simulink model "Part1_Developing_a_Vehicle_Model_in_Simulink_from_Scratch"  (R2021a)
settings: Solver=VariableStepAuto  StartTime=0.0  StopTime=10.0  RelTol=1e-3
settings Model: Creator=QZHAN112  LastModifiedBy=QZHAN112

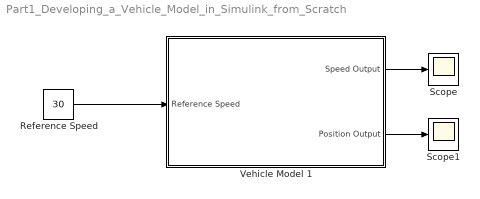
== system Part1_Developing_a_Vehicle_Model_in_Simulink_from_Scratch ==
  Reference Speed : Constant  Value=30
  Scope : Scope
  Scope1 : Scope
  Vehicle Model 1 : Subsystem  mask{Pos=100, Speed=20}
      mask prompts: Pos "Initial Position"; Speed "Initial Speed"
      mask TypeOptions Pos: Initial Position/Value
      mask TypeOptions Speed: Initial Speed/Value
      mask Display: image('model-based autonomous traffic simulation framework\Toyota.gif');
  wires:
  Vehicle Model 1/1(Speed Output) -> Scope/1
  Vehicle Model 1/2(Position Output) -> Scope1/1
  Reference Speed/1 -> Vehicle Model 1/1(Reference Speed)

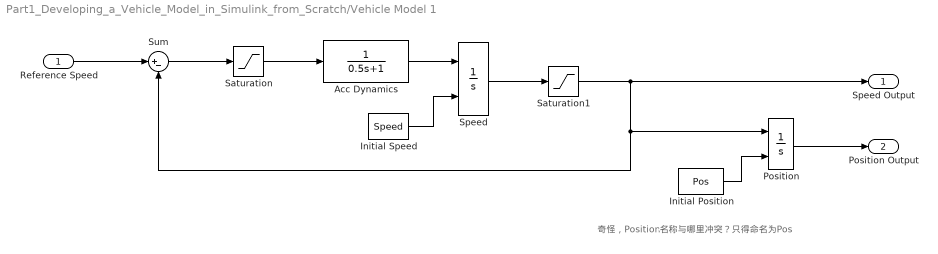
== system Part1_Developing_a_Vehicle_Model_in_Simulink_from_Scratch/Vehicle Model 1 ==
  note: 奇怪，Position名称与哪里冲突？只得命名为Pos
  Reference Speed : Inport
  Acc Dynamics : TransferFcn  Denominator=[0.5 1]
  Initial Position : Constant  Value=Pos
  Initial Speed : Constant  Value=Speed
  Position : Integrator  InitialConditionSource=external
  Saturation : Saturate  UpperLimit=2  LowerLimit=-3
  Saturation1 : Saturate  UpperLimit=inf  LowerLimit=0
  Speed : Integrator  InitialConditionSource=external
  Sum : Sum  Inputs=|+-
  Speed Output : Outport
  Position Output : Outport  Port=2
  wires:
  Saturation/1 -> Acc Dynamics/1
  Acc Dynamics/1 -> Speed/1
  Speed/1 -> Saturation1/1
  Position/1 -> Position Output/1
  Saturation1/1 -> Speed Output/1, Sum/2, Position/1
  Reference Speed/1 -> Sum/1
  Initial Speed/1 -> Speed/2
  Sum/1 -> Saturation/1
  Initial Position/1 -> Position/2
